simulink model "mpc_forces"  (R2018b)
settings: Solver=FixedStepDiscrete  StartTime=0.0  StopTime=Tstop  FixedStep=Ts  RelTol=1e-3  EnableMultiTasking=on
values from neighbouring files (symbols this model uses):
  p = 3    [forcesmpc_timevarying.m]
  Ts = 0.1    [forcesmpc_timevarying.m]
  Tstop = 25    [forcesmpc_timevarying.m]
  x0 = zeros(nx, 1)    [forcesmpc_timevarying.m]
libraries: forceslib x3
settings Model: Creator=The MathWorks, Inc.  LastModifiedBy=NivethanYogarajah
settings DataIOCC: LimitDataPoints=on
settings OptimizationCC: LifeSpan=inf
settings DebuggingCC: AllowSymbolicDim=off  SFUnexpectedBacktrackingDiag=warning  SFNoUnconditionalDefaultTransitionDiag=warning  SFExecutionAtInitializationDiag=none
settings ModelReferenceCC: PropagateSignalLabelsOutOfModel=off
settings SFSimCC: SimUseLocalCustomCode=off
settings RTWCC: RTWUseLocalCustomCode=off
settings CodeAppCC: StateflowObjectComments=on
settings GRTTargetCC: TargetLangStandard=C89/C90 (ANSI)
settings ConfigComp: CovMetricSettings=dw  CovSaveCumulativeToWorkspaceVar=on  CovSaveSingleToWorkspaceVar=on  CovExternalEMLEnable=off

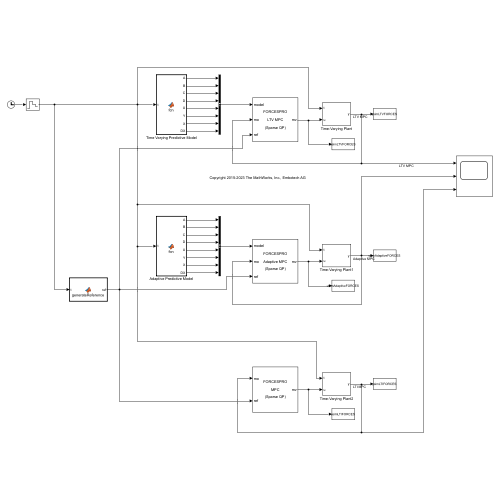
[thumbnail: Simulink's stored preview of the top-level diagram]
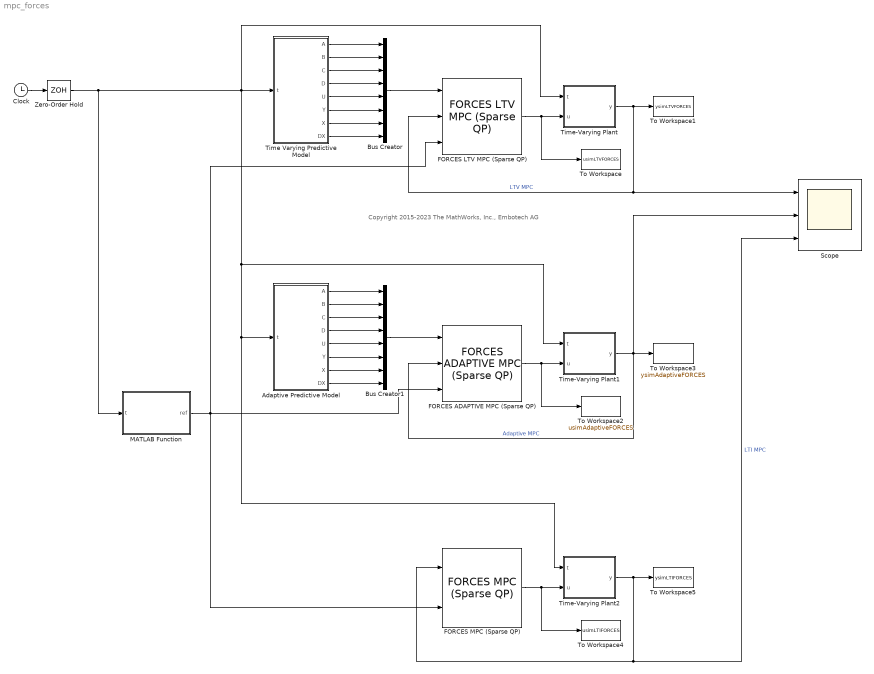
== system mpc_forces ==
  note: Copyright 2015-2023 The MathWorks, Inc., Embotech AG
  Adaptive Predictive Model : MATLAB Function  TreatAsAtomicUnit=on
  Bus Creator : BusCreator  Inputs=8
  Bus Creator1 : BusCreator  Inputs=8
  Clock : Clock
  FORCES ADAPTIVE MPC (Sparse QP) : forceslib/FORCES ADAPTIVE MPC (Sparse QP)  CoreData=coredataAdaptive  StateData=statedataAdaptive  md_inport=off  mv_inport=off  uref_inport=off  state_inport=off  ymin_inport=off  ymax_inport=off  umin_inport=off  umax_inport=off  dumin_inport=off  dumax_inport=off  ywt_inport=off  uwt_inport=off  duwt_inport=off  ecrwt_inport=off  return_cost=off  return_mvseq=off  return_qpstatus=off  return_qpsolvetime=off  return_solverid=off  return_xseq=off  return_state=off  return_yseq=off
      settings: SourceProductName=FORCESPRO MPC Blocks
  FORCES LTV MPC (Sparse QP) : forceslib/FORCES LTV MPC (Sparse QP)  CoreData=coredataLTV  StateData=statedataLTV  md_inport=off  mv_inport=off  uref_inport=off  state_inport=off  ymin_inport=off  ymax_inport=off  umin_inport=off  umax_inport=off  dumin_inport=off  dumax_inport=off  ywt_inport=off  uwt_inport=off  duwt_inport=off  ecrwt_inport=off  return_cost=off  return_mvseq=off  return_qpstatus=off  return_qpsolvetime=off  return_solverid=off  return_xseq=off  return_state=off  return_yseq=off
      settings: SourceProductName=FORCESPRO MPC Blocks
  FORCES MPC (Sparse QP) : forceslib/FORCES MPC (Sparse QP)  CoreData=coredataLTI  StateData=statedataLTI  md_inport=off  mv_inport=off  uref_inport=off  state_inport=off  ymin_inport=off  ymax_inport=off  umin_inport=off  umax_inport=off  dumin_inport=off  dumax_inport=off  ywt_inport=off  uwt_inport=off  duwt_inport=off  ecrwt_inport=off  return_cost=off  return_mvseq=off  return_qpstatus=off  return_qpsolvetime=off  return_solverid=off  return_xseq=off  return_state=off  return_yseq=off
      settings: SourceProductName=FORCESPRO MPC Blocks
  MATLAB Function : MATLAB Function  TreatAsAtomicUnit=on
  Scope : Scope  NumInputPorts=3
  Time Varying Predictive Model : MATLAB Function  TreatAsAtomicUnit=on
  Time-Varying Plant : Subsystem
  Time-Varying Plant1 : Subsystem
  Time-Varying Plant2 : Subsystem
  To Workspace : ToWorkspace  VariableName=usimLTVFORCES  SampleTime=-1
  To Workspace1 : ToWorkspace  VariableName=ysimLTVFORCES  SampleTime=-1
  To Workspace2 : ToWorkspace  VariableName=usimAdaptiveFORCES  SampleTime=-1
  To Workspace3 : ToWorkspace  VariableName=ysimAdaptiveFORCES  SampleTime=-1
  To Workspace4 : ToWorkspace  VariableName=usimLTIFORCES  SampleTime=-1
  To Workspace5 : ToWorkspace  VariableName=ysimLTIFORCES  SampleTime=-1
  Zero-Order Hold : ZeroOrderHold  SampleTime=Ts
  wires:
  Clock/1 -> Zero-Order Hold/1
  Time Varying Predictive Model/1(A) -> Bus Creator/1
  Time Varying Predictive Model/2(B) -> Bus Creator/2
  Time Varying Predictive Model/3(C) -> Bus Creator/3
  Time Varying Predictive Model/5(U) -> Bus Creator/5
  Time Varying Predictive Model/6(Y) -> Bus Creator/6
  Time Varying Predictive Model/7(X) -> Bus Creator/7
  Time Varying Predictive Model/8(DX) -> Bus Creator/8
  Time Varying Predictive Model/4(D) -> Bus Creator/4
  Bus Creator/1 -> FORCES LTV MPC (Sparse QP)/1
  FORCES LTV MPC (Sparse QP)/1 -> To Workspace/1, Time-Varying Plant/2(u)
  Zero-Order Hold/1 -> MATLAB Function/1(t), Time-Varying Plant/1(t), Time Varying Predictive Model/1(t), Time-Varying Plant1/1(t), Adaptive Predictive Model/1(t), Time-Varying Plant2/1(t)
  Time-Varying Plant/1(y) -> FORCES LTV MPC (Sparse QP)/2, Scope/1, To Workspace1/1  "LTV MPC"
  Adaptive Predictive Model/6(Y) -> Bus Creator1/6
  Adaptive Predictive Model/5(U) -> Bus Creator1/5
  Time-Varying Plant1/1(y) -> FORCES ADAPTIVE MPC (Sparse QP)/2, Scope/2, To Workspace3/1  "Adaptive MPC"
  Adaptive Predictive Model/3(C) -> Bus Creator1/3
  Bus Creator1/1 -> FORCES ADAPTIVE MPC (Sparse QP)/1
  Adaptive Predictive Model/1(A) -> Bus Creator1/1
  Adaptive Predictive Model/4(D) -> Bus Creator1/4
  FORCES ADAPTIVE MPC (Sparse QP)/1 -> To Workspace2/1, Time-Varying Plant1/2(u)
  Adaptive Predictive Model/7(X) -> Bus Creator1/7
  Adaptive Predictive Model/8(DX) -> Bus Creator1/8
  Adaptive Predictive Model/2(B) -> Bus Creator1/2
  FORCES MPC (Sparse QP)/1 -> To Workspace4/1, Time-Varying Plant2/2(u)
  Time-Varying Plant2/1(y) -> FORCES MPC (Sparse QP)/1, Scope/3, To Workspace5/1  "LTI MPC"
  MATLAB Function/1(ref) -> FORCES MPC (Sparse QP)/2, FORCES LTV MPC (Sparse QP)/3, FORCES ADAPTIVE MPC (Sparse QP)/3

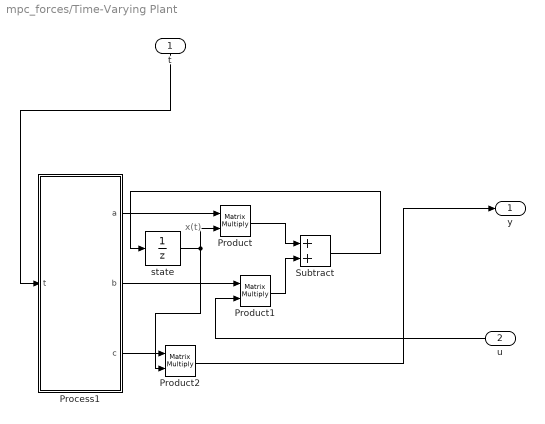
== system mpc_forces/Time-Varying Plant ==
  note: x(t)
  t : Inport
  u : Inport  Port=2
  Process1 : MATLAB Function  TreatAsAtomicUnit=on  SystemSampleTime=Ts
  Product : Product  Multiplication=Matrix(*)
  Product1 : Product  Multiplication=Matrix(*)
  Product2 : Product  Multiplication=Matrix(*)
  Subtract : Sum
  state : UnitDelay  InitialCondition=x0  SampleTime=Ts  HasFrameUpgradeWarning=on
  y : Outport
  wires:
  Process1/1(a) -> Product/1
  Product2/1 -> y/1
  Product/1 -> Subtract/1
  Product1/1 -> Subtract/2
  Process1/2(b) -> Product1/1
  u/1 -> Product1/2
  t/1 -> Process1/1(t)
  Process1/3(c) -> Product2/1
  state/1 -> Product/2, Product2/2
  Subtract/1 -> state/1

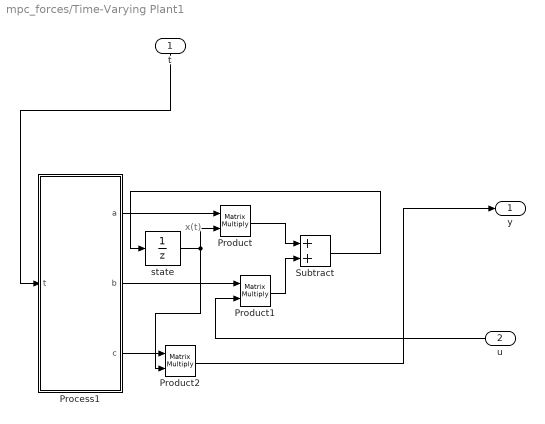
== system mpc_forces/Time-Varying Plant1 ==
  note: x(t)
  t : Inport
  u : Inport  Port=2
  Process1 : MATLAB Function  TreatAsAtomicUnit=on  SystemSampleTime=Ts
  Product : Product  Multiplication=Matrix(*)
  Product1 : Product  Multiplication=Matrix(*)
  Product2 : Product  Multiplication=Matrix(*)
  Subtract : Sum
  state : UnitDelay  InitialCondition=x0  SampleTime=Ts  HasFrameUpgradeWarning=on
  y : Outport
  wires:
  Process1/1(a) -> Product/1
  Product2/1 -> y/1
  Product/1 -> Subtract/1
  Product1/1 -> Subtract/2
  Process1/2(b) -> Product1/1
  u/1 -> Product1/2
  t/1 -> Process1/1(t)
  Process1/3(c) -> Product2/1
  state/1 -> Product/2, Product2/2
  Subtract/1 -> state/1

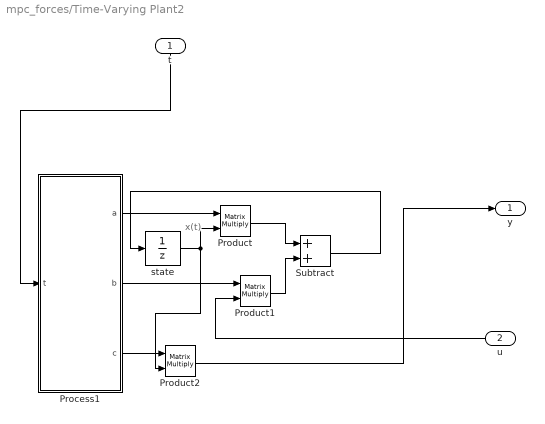
== system mpc_forces/Time-Varying Plant2 ==
  note: x(t)
  t : Inport
  u : Inport  Port=2
  Process1 : MATLAB Function  TreatAsAtomicUnit=on  SystemSampleTime=Ts
  Product : Product  Multiplication=Matrix(*)
  Product1 : Product  Multiplication=Matrix(*)
  Product2 : Product  Multiplication=Matrix(*)
  Subtract : Sum
  state : UnitDelay  InitialCondition=x0  SampleTime=Ts  HasFrameUpgradeWarning=on
  y : Outport
  wires:
  Process1/1(a) -> Product/1
  Product2/1 -> y/1
  Product/1 -> Subtract/1
  Product1/1 -> Subtract/2
  Process1/2(b) -> Product1/1
  u/1 -> Product1/2
  t/1 -> Process1/1(t)
  Process1/3(c) -> Product2/1
  state/1 -> Product/2, Product2/2
  Subtract/1 -> state/1

== matlab function mpc_forces/Time Varying Predictive Model ==
  data: t input; Ts parameter; A output; B output; C output; D output; U output; Y output; X output; DX output; p parameter
function [A,B,C,D,U,Y,X,DX] = fcn(t,Ts,p)
%#codegen

coder.extrinsic('ss');
coder.extrinsic('c2d');
coder.extrinsic('tf');
coder.extrinsic('ssdata');

nx=3; % number of states

A=zeros(nx,nx,p+1);
B=zeros(nx,1,p+1);
C=zeros(1,nx,p+1);
D=zeros(1,1,p+1);
U=zeros(1,1,p+1);
Y=zeros(1,1,p+1);
X=zeros(nx,1,p+1);
DX=zeros(nx,1,p+1);

for k=0:p
    [a,b,c,d]=ssdata(ss(c2d(tf([5 5+2*cos((t/Ts+k)/4)],[1 3 2 6+1*sin((t/Ts+k)/2)]),Ts)));
     A(:,:,k+1)=a;
     B(:,:,k+1)=b;
     C(:,:,k+1)=c;
     D(:,:,k+1)=d;
     U(:,:,k+1)=0;
     Y(:,:,k+1)=0;
     X(:,:,k+1)=zeros(nx,1);
     DX(:,:,k+1)=zeros(nx,1);
end

== matlab function mpc_forces/Time-Varying Plant/Process1 ==
  data: a output; b output; t input; c output; Ts parameter
function [a,b,c] = fcn(t,Ts)
%#codegen

coder.extrinsic('ss');
coder.extrinsic('c2d');
coder.extrinsic('tf');
coder.extrinsic('ssdata');

nx=3;
a=zeros(nx,nx);
b=zeros(nx,1);
c=zeros(1,nx);

[a,b,c]=ssdata(ss(c2d(tf([5 5+2*cos(t/Ts/4)],[1 3 2 6+1*sin(t/Ts/2)]),Ts)));

== matlab function mpc_forces/Adaptive Predictive Model ==
  data: t input; Ts parameter; A output; B output size=[3, 1]; C output size=[1, 3]; D output size=[1, 1]; U output size=[1, 1]; Y output size=[1, 1]; X output size=[3, 1]; DX output size=[3, 1]
function [A,B,C,D,U,Y,X,DX] = fcn(t,Ts)
%#codegen

coder.extrinsic('ss');
coder.extrinsic('c2d');
coder.extrinsic('tf');
coder.extrinsic('ssdata');

nx = 3; % number of states
A = zeros(nx, nx);
B = zeros(nx, 1);
C = zeros(1, nx);
D = zeros(1, 1);
U = zeros(1, 1);
Y = zeros(1, 1);
X = zeros(nx, 1);
DX = zeros(nx, 1);

k = 0;
[A(:), B(:), C(:), D(:)] = ssdata(ss(c2d(tf([5 5+2*cos((t/Ts+k)/4)],[1 3 2 6+1*sin((t/Ts+k)/2)]),Ts)));
 U(:) = 0;
 Y(:) = 0;
 X(:) = zeros(nx,1);
 DX(:) = zeros(nx,1);

== matlab function mpc_forces/Time-Varying Plant1/Process1 ==
  data: a output; b output; t input; c output; Ts parameter
function [a,b,c] = fcn(t,Ts)
%#codegen

coder.extrinsic('ss');
coder.extrinsic('c2d');
coder.extrinsic('tf');
coder.extrinsic('ssdata');

nx=3;
a=zeros(nx,nx);
b=zeros(nx,1);
c=zeros(1,nx);

[a,b,c]=ssdata(ss(c2d(tf([5 5+2*cos(t/Ts/4)],[1 3 2 6+1*sin(t/Ts/2)]),Ts)));

== matlab function mpc_forces/MATLAB Function ==
  data: t input; ref output; Ts parameter; Tstop parameter
function ref = generateReference(t, Ts, Tstop)
    p=3;
    Nsim = round(Tstop/Ts) + 1;

    stepSwitch = round(Nsim/3);
    references = ones(Nsim+p, 1);
    references(stepSwitch:2*stepSwitch-1) = 0.6;
    references(2*stepSwitch:end) = 0.25;
    
    ct = round(t/Ts) + 1;
    ref = zeros(p,1);
    ref(:) = references(ct:ct+p-1);
end

== matlab function mpc_forces/Time-Varying Plant2/Process1 ==
  data: a output; b output; t input; c output; Ts parameter
function [a,b,c] = fcn(t,Ts)
%#codegen

coder.extrinsic('ss');
coder.extrinsic('c2d');
coder.extrinsic('tf');
coder.extrinsic('ssdata');

nx=3;
a=zeros(nx,nx);
b=zeros(nx,1);
c=zeros(1,nx);

[a,b,c]=ssdata(ss(c2d(tf([5 5+2*cos(t/Ts/4)],[1 3 2 6+1*sin(t/Ts/2)]),Ts)));
